simulink library "twoNodeTether_cl"  (R2018b)
settings: Solver=VariableStepAuto  StartTime=0.0  StopTime=10.0  RelTol=1e-3
undefined symbols (not defined in the file or in its folder): fluidDensity, gravity, thrStructure
libraries: nodeDragForce_ul x1, nodeNetBuoyForce_ul x1, nodePosToLinkPos_ul x1, nodeSpringDamperForce_ul x1
settings Model: Creator=mcobb  LastModifiedBy=mitch

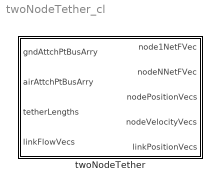
== system twoNodeTether_cl ==
  twoNodeTether : Subsystem  VariantControl=twoNodeTether  mask{thr=thrStructure, flowDensity=fluidDensity, gravity=gravity}
      mask prompts: thr "Tether Structure"; flowDensity "Fluid Density"; gravity "Gravitational Acceleration"

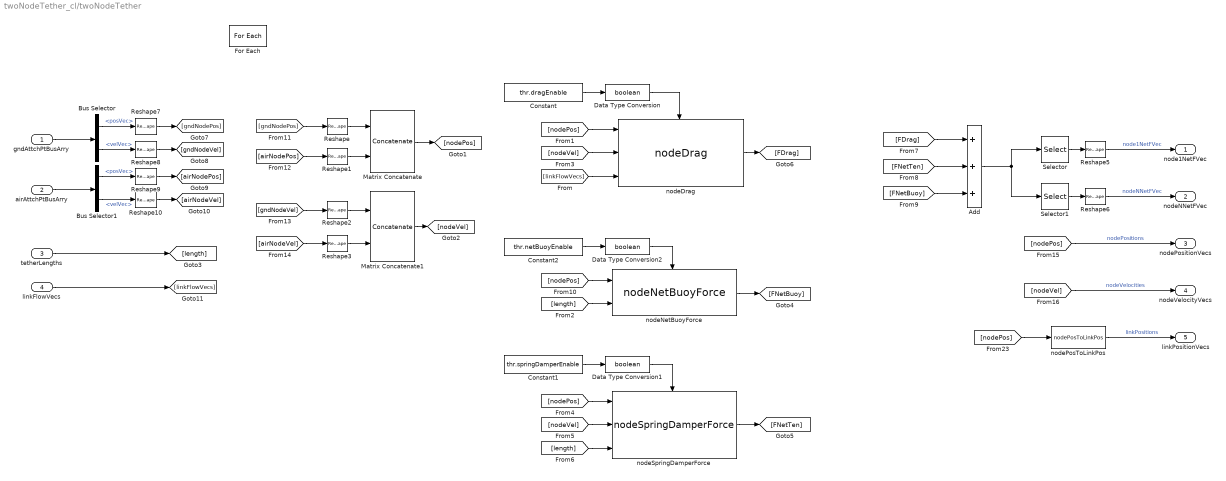
== system twoNodeTether_cl/twoNodeTether ==
  gndAttchPtBusArry : Inport  OutDataTypeStr=Bus: thrAttachPtKinematicsBus  Partition=on  PartitionDimension=1  PartitionWidth=1  PartitionOffset=0
  airAttchPtBusArry : Inport  Port=2  OutDataTypeStr=Bus: thrAttachPtKinematicsBus  Partition=on  PartitionDimension=1  PartitionWidth=1  PartitionOffset=0
  tetherLengths : Inport  Port=3  Partition=on  PartitionDimension=1  PartitionWidth=1  PartitionOffset=0
  linkFlowVecs : Inport  Port=4  Partition=on  PartitionDimension=3  PartitionWidth=1  PartitionOffset=0
  Add : Sum  Inputs=3
  Bus Selector : BusSelector  OutputSignals=posVec,velVec
  Bus Selector1 : BusSelector  OutputSignals=posVec,velVec
  Constant : Constant  Value=thr.dragEnable
  Constant1 : Constant  Value=thr.springDamperEnable
  Constant2 : Constant  Value=thr.netBuoyEnable
  Data Type Conversion : DataTypeConversion  OutDataTypeStr=boolean
  Data Type Conversion1 : DataTypeConversion  OutDataTypeStr=boolean
  Data Type Conversion2 : DataTypeConversion  OutDataTypeStr=boolean
  For Each : ForEach  DisableCoverage=on  IterateSubsysMaskParameter=on,off,off  SubsysMaskParameterIterationDimension=2,1,1  IndexMode=One-based
  Matrix Concatenate : Concatenate  Mode=Multidimensional array  ConcatenateDimension=2
  Matrix Concatenate1 : Concatenate  Mode=Multidimensional array  ConcatenateDimension=2
  Reshape{,1..3,5..10} (10 alike) : Reshape  OutputDimensionality=Column vector (2-D)
  Selector : Selector  NumberOfDimensions=2  InputPortWidth=3  IndexOptions=Select all,Index vector (dialog)  Indices=[1 3],1  OutputSizes=1,1
  Selector1 : Selector  NumberOfDimensions=2  InputPortWidth=3  IndexOptions=Select all,Index vector (dialog)  Indices=[1 3],2  OutputSizes=1,1
  nodeDrag : nodeDragForce_ul/nodeDrag  flowDensity=flowDensity  thrDiam=thr.diameter  dragCoeff=thr.dragCoeff
  nodeNetBuoyForce : nodeNetBuoyForce_ul/nodeNetBuoyForce  fluidDensity=flowDensity  tetherDensity=thr.density  diameter=thr.diameter  gravity=gravity
  nodePosToLinkPos : nodePosToLinkPos_ul/nodePosToLinkPos  SystemSampleTime=-1
  nodeSpringDamperForce : nodeSpringDamperForce_ul/nodeSpringDamperForce  mass=thr.vehicleMass  zeta=thr.dampingRatio  diameter=thr.diameter  youngsMod=thr.youngsMod
  node1NetFVec : Outport  ConcatenationDimension=3
  nodeNNetFVec : Outport  Port=2  ConcatenationDimension=3
  nodePositionVecs : Outport  Port=3  ConcatenationDimension=3
  nodeVelocityVecs : Outport  Port=4  ConcatenationDimension=3
  linkPositionVecs : Outport  Port=5  ConcatenationDimension=3
  wires:
  [linkFlowVecs] -> nodeDrag/3
  [nodeVel] -> nodeDrag/2
  [gndNodePos] -> Reshape/1
  [gndNodeVel] -> Reshape2/1
  [airNodePos] -> Reshape1/1
  [airNodeVel] -> Reshape3/1
  Reshape/1 -> Matrix Concatenate/1
  Reshape1/1 -> Matrix Concatenate/2
  Reshape3/1 -> Matrix Concatenate1/2
  Reshape2/1 -> Matrix Concatenate1/1
  Matrix Concatenate/1 -> [nodePos]
  [nodePos] -> nodeDrag/1
  tetherLengths/1 -> [length]
  [length] -> nodeNetBuoyForce/2
  [nodeVel] -> nodeSpringDamperForce/2
  [nodePos] -> nodeSpringDamperForce/1
  [length] -> nodeSpringDamperForce/3
  nodeNetBuoyForce/1 -> [FNetBuoy]
  nodeSpringDamperForce/1 -> [FNetTen]
  nodeDrag/1 -> [FDrag]
  [FNetTen] -> Add/2
  [FDrag] -> Add/1
  [FNetBuoy] -> Add/3
  Selector/1 -> Reshape5/1
  Add/1 -> Selector1/1, Selector/1
  Selector1/1 -> Reshape6/1
  [nodePos] -> nodeNetBuoyForce/1
  Matrix Concatenate1/1 -> [nodeVel]
  Bus Selector/1 -> Reshape7/1  "<posVec>"
  gndAttchPtBusArry/1 -> Bus Selector/1
  Bus Selector/2 -> Reshape8/1  "<velVec>"
  Bus Selector1/2 -> Reshape10/1  "<velVec>"
  airAttchPtBusArry/1 -> Bus Selector1/1
  Bus Selector1/1 -> Reshape9/1  "<posVec>"
  Reshape7/1 -> [gndNodePos]
  Reshape8/1 -> [gndNodeVel]
  Reshape9/1 -> [airNodePos]
  Reshape10/1 -> [airNodeVel]
  Constant/1 -> Data Type Conversion/1
  Data Type Conversion/1 -> nodeDrag/Enable
  Data Type Conversion1/1 -> nodeSpringDamperForce/Enable
  Constant1/1 -> Data Type Conversion1/1
  Constant2/1 -> Data Type Conversion2/1
  Data Type Conversion2/1 -> nodeNetBuoyForce/Enable
  [nodePos] -> nodePosToLinkPos/1
  linkFlowVecs/1 -> [linkFlowVecs]
  nodePosToLinkPos/1 -> linkPositionVecs/1  "linkPositions"
  [nodeVel] -> nodeVelocityVecs/1  "nodeVelocities"
  [nodePos] -> nodePositionVecs/1  "nodePositions"
  Reshape5/1 -> node1NetFVec/1  "node1NetFVec"
  Reshape6/1 -> nodeNNetFVec/1  "nodeNNetFVec"
